simulink subsystem "SCIInAbstractionFocQep"  (R2024a)
settings: Solver=VariableStepAuto  StartTime=0.0  StopTime=10.0  RelTol=1e-3
libraries: simulink x2
settings Model: Creator=The MathWorks, Inc.  LastModifiedBy=snarayan
settings RTWCC: GPUComputeCapability=3.5

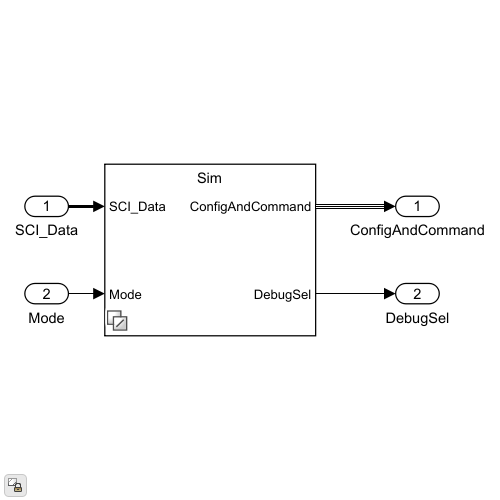
[thumbnail: Simulink's stored preview of the top-level diagram]
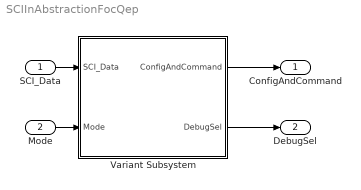
== system SCIInAbstractionFocQep ==
  SCI_Data : Inport
  Mode : Inport  Port=2
  Variant Subsystem : Subsystem  Variant=on  VariantControlMode=sim codegen switching
  ConfigAndCommand : Outport
  DebugSel : Outport  Port=2
  wires:
  SCI_Data/1 -> Variant Subsystem/1(SCI_Data)
  Variant Subsystem/2(DebugSel) -> DebugSel/1
  Variant Subsystem/1(ConfigAndCommand) -> ConfigAndCommand/1
  Mode/1 -> Variant Subsystem/2(Mode)

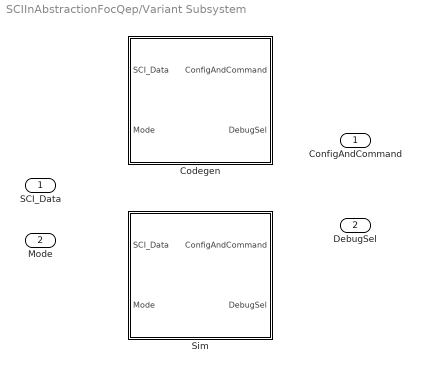
== system SCIInAbstractionFocQep/Variant Subsystem ==
  SCI_Data : Inport
  Mode : Inport  Port=2
  Codegen : Subsystem  VariantControl=(codegen)
  Sim : Subsystem  VariantControl=(sim)
  ConfigAndCommand : Outport
  DebugSel : Outport  Port=2

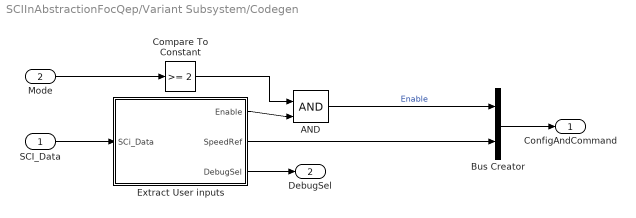
== system SCIInAbstractionFocQep/Variant Subsystem/Codegen ==
  SCI_Data : Inport
  Mode : Inport  Port=2
  AND : Logic  IconShape=distinctive  AllPortsSameDT=off  OutDataTypeStr=boolean
  Bus Creator : BusCreator  Inputs=2
  Compare To Constant : simulink/Logic and Bit Operations/Compare To Constant  relop=>=  const=2  OutDataTypeStr=boolean
  Extract User inputs : Subsystem
  ConfigAndCommand : Outport
  DebugSel : Outport  Port=2
  wires:
  Extract User inputs/1(Enable) -> AND/2
  Compare To Constant/1 -> AND/1
  Extract User inputs/2(SpeedRef) -> Bus Creator/2
  Mode/1 -> Compare To Constant/1
  Extract User inputs/3(DebugSel) -> DebugSel/1
  SCI_Data/1 -> Extract User inputs/1(SCi_Data)
  AND/1 -> Bus Creator/1  "Enable"
  Bus Creator/1 -> ConfigAndCommand/1

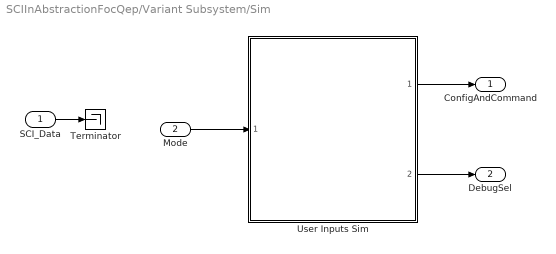
== system SCIInAbstractionFocQep/Variant Subsystem/Sim ==
  SCI_Data : Inport
  Mode : Inport  Port=2
  Terminator : Terminator
  User Inputs Sim : Subsystem  ReferencedSubsystem=SystemInputsSimFocQep
  ConfigAndCommand : Outport
  DebugSel : Outport  Port=2
  wires:
  User Inputs Sim/2 -> DebugSel/1
  User Inputs Sim/1 -> ConfigAndCommand/1
  Mode/1 -> User Inputs Sim/1
  SCI_Data/1 -> Terminator/1

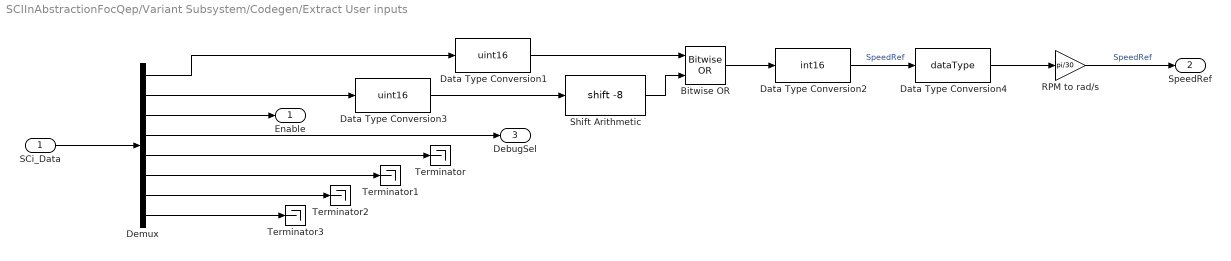
== system SCIInAbstractionFocQep/Variant Subsystem/Codegen/Extract User inputs ==
  SCi_Data : Inport
  Bitwise OR : simulink/Logic and Bit Operations/Bitwise Operator  logicop=OR  UseBitMask=off  NumInputPorts=2  BitMask=bin2dec('11011001')  BitMaskRealWorld=Stored Integer
      settings: LibrarySourceBlock=|
      | simulink/Quick Insert/Logic and Bit
      | Operations/Bitwise OR
  Data Type Conversion1 : DataTypeConversion  OutDataTypeStr=uint16  RndMeth=Simplest  SaturateOnIntegerOverflow=off
  Data Type Conversion2 : DataTypeConversion  OutDataTypeStr=int16  ConvertRealWorld=Stored Integer (SI)  RndMeth=Simplest  SaturateOnIntegerOverflow=off
  Data Type Conversion3 : DataTypeConversion  OutDataTypeStr=uint16  RndMeth=Simplest  SaturateOnIntegerOverflow=off
  Data Type Conversion4 : DataTypeConversion  OutDataTypeStr=dataType  RndMeth=Simplest  SaturateOnIntegerOverflow=off
  Demux : Demux  Outputs=8
  RPM to rad/s : Gain  Gain=pi/30  RndMeth=Simplest  OutDataTypeStr=Inherit: Same as input
  Shift Arithmetic : ArithShift  BitShiftNumber=-8
  Terminator{,1..3} (4 alike) : Terminator
  Enable : Outport
  SpeedRef : Outport  Port=2
  DebugSel : Outport  Port=3
  wires:
  Data Type Conversion4/1 -> RPM to rad/s/1
  RPM to rad/s/1 -> SpeedRef/1  "SpeedRef"
  Demux/8 -> Terminator3/1
  Demux/6 -> Terminator1/1
  Demux/5 -> Terminator/1
  Demux/2 -> Data Type Conversion3/1
  Demux/7 -> Terminator2/1
  Data Type Conversion1/1 -> Bitwise OR/1
  Data Type Conversion3/1 -> Shift Arithmetic/1
  Shift Arithmetic/1 -> Bitwise OR/2
  SCi_Data/1 -> Demux/1
  Demux/1 -> Data Type Conversion1/1
  Bitwise OR/1 -> Data Type Conversion2/1
  Demux/4 -> DebugSel/1
  Data Type Conversion2/1 -> Data Type Conversion4/1  "SpeedRef"
  Demux/3 -> Enable/1
